simulink subsystem "Cathode_Simscape_ControllerWrapper_RefSub"  (R2023a)
settings: Solver=VariableStepAuto  StartTime=0.0  StopTime=10.0  RelTol=1e-3
undefined symbols (not defined in the file or in its folder): CAC_STATE, init_Parameters, struct_OMM_Set, struct_Sensors
libraries: simulink x1
settings Model: Creator=daniel.mead  LastModifiedBy=daniel.mead

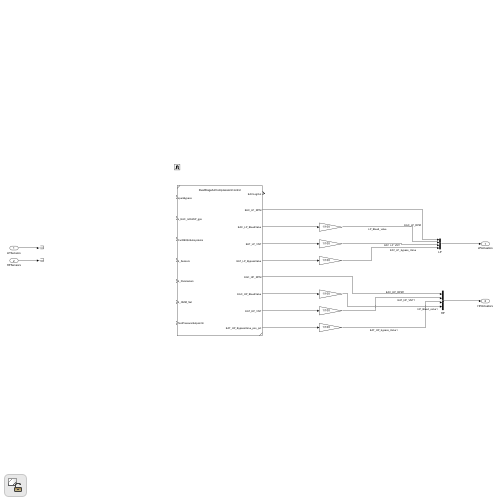
[thumbnail: Simulink's stored preview of the top-level diagram]
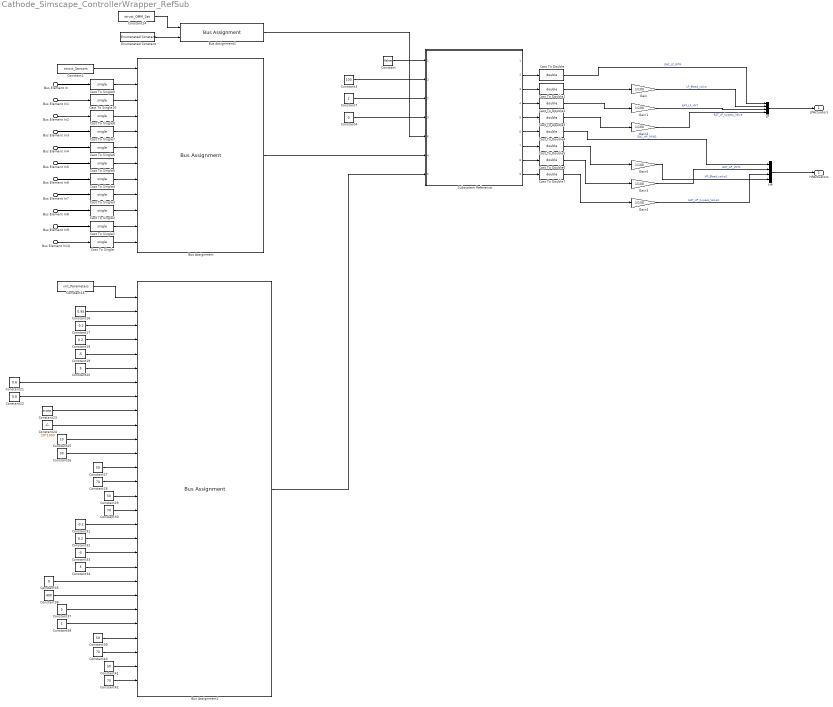
== system Cathode_Simscape_ControllerWrapper_RefSub ==
  Bus Element In : Inport  PortName=Sensors  Element=FT-C001
  Bus Element In1 : Inport  PortName=Sensors  Element=PT-C-001
  Bus Element In2 : Inport  PortName=Sensors  Element=TT-C-001
  Bus Element In3 : Inport  PortName=Sensors  Element=PT701
  Bus Element In4 : Inport  PortName=Sensors  Element=PT721
  Bus Element In5 : Inport  PortName=Sensors  Element=PT-C-201
  Bus Element In6 : Inport  PortName=Sensors  Element=PT-C-411
  Bus Element In7 : Inport  PortName=Sensors  Element=FT-C-201
  Bus Element In8 : Inport  PortName=Sensors  Element=PT-C-211
  Bus Element In9 : Inport  PortName=Sensors  Element=TT-C-201
  Bus Element In10 : Inport  PortName=Sensors  Element=FT-C-411
  Bus Assignment : BusAssignment  AssignedSignals=b_CathodeSens.b_Sens_SystemInlet.FTC001_mDot_gps_get,b_CathodeSens.b_Sens_SystemInlet.PTC001_p_bara_get,b_CathodeSens.b_Sens_SystemInlet.TTC001_T_degC_get,b_CathodeSens.b_Sens_EAT_LP_Inlet.PTC701_p_bara_get,b_CathodeSens.b_Sens_SystemOutlet.PTC721_p_bara_get,b_CathodeSens.b_Sens_EAC_HP_Inlet.PTC201_p_bara_get,b_CathodeSens.b_Sens_StackInlet.PTC411_p_bara_get,b_CathodeSens.b_Sens_EAC_HP_Inlet.FTC201_mDot_gps_get,b_CathodeSens.b_Sens_EAC_HP_Outlet.PTC211_p_bara_get,b_CathodeSens.b_Sens_EAC_HP_Inlet.TTC201_T_degC_get,b_CathodeSens.b_Sens_HumInlet.FTC321_mDot_gps_get
  Bus Assignment1 : BusAssignment  AssignedSignals=b_OMM_Cathode_Set.s_CAC_StateSetREQ_enum
  Bus Assignment2 : BusAssignment  AssignedSignals=b_CAT_Parameters.b_CAC_Parameters.DSACLP_TH_AdverseRatioStopValve,b_CAT_Parameters.b_CAC_Parameters.DSACLP_LRL_EATpCtrlSurProtSPChng,b_CAT_Parameters.b_CAC_Parameters.DSACLP_URL_EATpCtrlSurProtSPChng,b_CAT_Parameters.b_CAC_Parameters.DSACLP_LRL_EACBleedSurProtSPChng,b_CAT_Parameters.b_CAC_Parameters.DSACLP_URL_EACBleedSurProtSPChng,b_CAT_Parameters.b_CAC_Parameters.DSACLP_P_PRallocation_pct,b_CAT_Parameters.b_CAC_Parameters.DSACLP_P_EATpSetMarginFactor,b_CAT_Parameters.b_CAC_Parameters.DSACLP_PID_PRcontrolEACRPM_P,b_CAT_Parameters.b_CAC_Parameters.DSACLP_PID_PRcontrolEACRPM_I,b_CAT_Parameters.b_CAC_Parameters.DSACLP_PID_PRcontrolEACBV_P,b_CAT_Parameters.b_CAC_Parameters.DSACLP_PID_PRcontrolEACBV_I,b_CAT_Parameters.b_CAC_Parameters.DSACLP_PID_pControlEATVNT_P,b_CAT_Parameters.b_CAC_Parameters.DSACLP_PID_pControlEATVNT_I,b_CAT_Parameters.b_CAC_Parameters.DSACLP_PID_pControlEATBV_P,b_CAT_Parameters.b_CAC_Parameters.DSACLP_PID_pControlEATBV_I,b_CAT_Parameters.b_CAC_Parameters.DSACHP_LRL_EATpCtrlSurProtSPChng,b_CAT_Parameters.b_CAC_Parameters.DSACHP_URL_EATpCtrlSurProtSPChng,b_CAT_Parameters.b_CAC_Parameters.DSACHP_LRL_EACBleedSurProtSPChng,b_CAT_Parameters.b_CAC_Parameters.DSACHP_URL_EACBleedSurProtSPChng,b_CAT_Parameters.b_CAC_Parameters.DSACHP_PID_mDotControlEACRPM_P,b_CAT_Parameters.b_CAC_Parameters.DSACHP_PID_mDotControlEACRPM_I,b_CAT_Parameters.b_CAC_Parameters.DSACHP_PID_mDotctrlEACBV_P,b_CAT_Parameters.b_CAC_Parameters.DSACHP_PID_mDotctrlEACBV_I,b_CAT_Parameters.b_CAC_Parameters.DSACHP_PID_pControlEATVNT_P,b_CAT_Parameters.b_CAC_Parameters.DSACHP_PID_pControlEATVNT_I,b_CAT_Parameters.b_CAC_Parameters.DSACHP_PID_pControlEATBV_P,b_CAT_Parameters.b_CAC_Parameters.DSACHP_PID_pControlEATBV_I
  Cast To Double{,1..7} (8 alike) : DataTypeConversion  OutDataTypeStr=double  SaturateOnIntegerOverflow=off  RndMeth=Floor
  Cast To Single{,1..10} (11 alike) : DataTypeConversion  OutDataTypeStr=single  SaturateOnIntegerOverflow=off  RndMeth=Floor
  Constant : Constant  Value=false  OutDataTypeStr=boolean
  Constant1 : Constant  Value=struct_Sensors  OutDataTypeStr=Bus: Sensors
  Constant14 : Constant  Value=struct_OMM_Set  OutDataTypeStr=Bus: OMM_Set
  Constant15 : Constant  Value=init_Parameters  OutDataTypeStr=Bus: Parameters
  Constant16 : Constant  Value=0.95  OutDataTypeStr=single
  Constant17 : Constant  Value=-0.2  OutDataTypeStr=single
  Constant18 : Constant  Value=0.2  OutDataTypeStr=single
  Constant19 : Constant  Value=-5  OutDataTypeStr=single
  Constant20 : Constant  Value=5  OutDataTypeStr=single
  Constant21 : Constant  Value=0.6  OutDataTypeStr=single
  Constant22 : Constant  Value=0.8  OutDataTypeStr=single
  Constant23 : Constant  Value=5*1000  OutDataTypeStr=single
  Constant24 : Constant  Value=20*1000  OutDataTypeStr=single
  Constant25 : Constant  Value=10  OutDataTypeStr=single
  Constant26 : Constant  Value=30  OutDataTypeStr=single
  Constant{27,29,39,41} (4 alike) : Constant  Value=50  OutDataTypeStr=single
  Constant{28,30,40,42} (4 alike) : Constant  Value=70  OutDataTypeStr=single
  Constant3 : Constant  Value=100  OutDataTypeStr=single
  Constant31 : Constant  Value=-0.2  OutDataTypeStr=single
  Constant32 : Constant  Value=0.2  OutDataTypeStr=single
  Constant33 : Constant  Value=-5  OutDataTypeStr=single
  Constant34 : Constant  Value=5  OutDataTypeStr=single
  Constant35 : Constant  Value=0  OutDataTypeStr=single
  Constant36 : Constant  Value=400  OutDataTypeStr=single
  Constant37 : Constant  Value=0  OutDataTypeStr=single
  Constant38 : Constant  OutDataTypeStr=single
  Constant4 : Constant  Value=0  OutDataTypeStr=single
  Constant7 : Constant  Value=2  OutDataTypeStr=single
  Enumerated Constant : simulink/Sources/Enumerated Constant  OutDataTypeStr=Enum: CAC_STATE  Value=CAC_STATE.Off  SampleTime=inf
  Gain{,1..5} (6 alike) : Gain  Gain=1/100
  HP : BusCreator  Inputs=4
  LP : BusCreator  Inputs=4
  Subsystem Reference : Subsystem  ReferencedSubsystem=DualStageAirCompressionControl
      settings: PortSchema="{\"entries\":[{\"content\":{\"sides\":[{\"content\":{\"connectorIds\":[\"In1\",\"In2\",\"In7\",\"In3\",\"In6\",\"In4\",\"In5\"]},\"type\":\"ConnectorPlacement.EquallySpacedRectSide\",\"uuid\":\"b5ba7dab-c5ac-4316-a132-05e487dafb7d\"},{\"content\":{\"connectorIds\":[\"Out1\",\"Out2\",\"Out3\",\"Out4\",\"Out5\",\"Out6\",\"Out7\",\"Out8\",\"Out9\"],\"side\":\"RIGHT\"},\"type\":\"ConnectorPlacement.EquallySpacedRectSide\",\"uuid\":\"c4904014-38e7-4722-936b-a5f9386463da\"},{\"content\":{\"side\":\"TOP\"},\"type\":\"ConnectorPlacement.EquallySpacedRectSide\",\"uuid\":\"115604c6-87d3-41ac-bea6-b4f46877a099\"}]},\"type\":\"ConnectorPlacement.EquallySpacedConnector\",\"uuid\":\"10366915-b484-482d-8f54-e3cd1476e2ec\"}],\"packageUris\":[\"http://schema.mathworks.com/mf0/Connector/R2020b\"],\"version\":\"1.0\"}"
  LPActuators : Outport
  HPActuators : Outport  Port=2
  wires:
  Gain4/1 -> HP/3  "EAT_HP_bypass_Valve1"
  Gain2/1 -> LP/4  "EAT_LP_bypass_Valve"
  Subsystem Reference/6 -> Cast To Double4/1
  Gain1/1 -> LP/3  "EAT_LP_VNT"
  Subsystem Reference/2 -> Cast To Double/1
  Gain5/1 -> HP/4  "HP_Bleed_valve1"
  Gain/1 -> LP/2  "LP_Bleed_valve"
  Gain3/1 -> HP/2  "EAT_HP_VNT1"
  LP/1 -> LPActuators/1
  HP/1 -> HPActuators/1
  Subsystem Reference/3 -> Cast To Double1/1
  Subsystem Reference/4 -> Cast To Double2/1
  Subsystem Reference/5 -> Cast To Double3/1
  Subsystem Reference/8 -> Cast To Double6/1
  Subsystem Reference/9 -> Cast To Double7/1
  Subsystem Reference/7 -> Cast To Double5/1
  Constant15/1 -> Bus Assignment2/1
  Constant34/1 -> Bus Assignment2/20
  Constant/1 -> Subsystem Reference/1
  Constant1/1 -> Bus Assignment/1
  Constant17/1 -> Bus Assignment2/3
  Constant39/1 -> Bus Assignment2/25
  Constant25/1 -> Bus Assignment2/11
  Constant42/1 -> Bus Assignment2/28
  Constant38/1 -> Bus Assignment2/24
  Constant35/1 -> Bus Assignment2/21
  Constant21/1 -> Bus Assignment2/7
  Constant32/1 -> Bus Assignment2/18
  Constant33/1 -> Bus Assignment2/19
  Constant23/1 -> Bus Assignment2/9
  Bus Assignment2/1 -> Subsystem Reference/5
  Constant28/1 -> Bus Assignment2/14
  Constant14/1 -> Bus Assignment1/1
  Bus Assignment/1 -> Subsystem Reference/4
  Constant31/1 -> Bus Assignment2/17
  Constant26/1 -> Bus Assignment2/12
  Constant37/1 -> Bus Assignment2/23
  Constant7/1 -> Subsystem Reference/7
  Constant30/1 -> Bus Assignment2/16
  Constant3/1 -> Subsystem Reference/2
  Constant16/1 -> Bus Assignment2/2
  Constant41/1 -> Bus Assignment2/27
  Constant40/1 -> Bus Assignment2/26
  Constant36/1 -> Bus Assignment2/22
  Constant29/1 -> Bus Assignment2/15
  Enumerated Constant/1 -> Bus Assignment1/2
  Bus Assignment1/1 -> Subsystem Reference/6
  Constant24/1 -> Bus Assignment2/10
  Constant27/1 -> Bus Assignment2/13
  Constant19/1 -> Bus Assignment2/5
  Constant22/1 -> Bus Assignment2/8
  Constant4/1 -> Subsystem Reference/3
  Constant20/1 -> Bus Assignment2/6
  Constant18/1 -> Bus Assignment2/4
  Bus Element In/1 -> Cast To Single9/1
  Bus Element In1/1 -> Cast To Single10/1
  Bus Element In2/1 -> Cast To Single8/1
  Bus Element In3/1 -> Cast To Single7/1
  Bus Element In4/1 -> Cast To Single6/1
  Bus Element In5/1 -> Cast To Single5/1
  Bus Element In6/1 -> Cast To Single4/1
  Bus Element In7/1 -> Cast To Single3/1
  Bus Element In8/1 -> Cast To Single2/1
  Bus Element In9/1 -> Cast To Single1/1
  Bus Element In10/1 -> Cast To Single/1
  Cast To Single/1 -> Bus Assignment/12
  Cast To Single1/1 -> Bus Assignment/11
  Cast To Single2/1 -> Bus Assignment/10
  Cast To Single3/1 -> Bus Assignment/9
  Cast To Single4/1 -> Bus Assignment/8
  Cast To Single5/1 -> Bus Assignment/7
  Cast To Single6/1 -> Bus Assignment/6
  Cast To Single7/1 -> Bus Assignment/5
  Cast To Single8/1 -> Bus Assignment/4
  Cast To Single10/1 -> Bus Assignment/3
  Cast To Single9/1 -> Bus Assignment/2
  Cast To Double/1 -> LP/1  "EAC_LP_RPM"
  Cast To Double1/1 -> Gain/1
  Cast To Double2/1 -> Gain1/1
  Cast To Double3/1 -> Gain2/1
  Cast To Double4/1 -> HP/1  "EAC_HP_RPM1"
  Cast To Double5/1 -> Gain5/1
  Cast To Double6/1 -> Gain3/1
  Cast To Double7/1 -> Gain4/1
